simulink model "Problem1"  (R2020b)
settings: Solver=VariableStepAuto  StartTime=0.0  StopTime=10.0  RelTol=1e-3
settings Model: Creator=HP  LastModifiedBy=HP

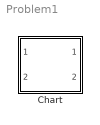
== system Problem1 ==
  Chart : Stateflow chart  TreatAsAtomicUnit=on

== stateflow chart Problem1/Chart ==
  state error
  state Coin_Inserted
  state Coke
  state Soda
  state Sprite
  state Pepsi
  (junction 5) -> error [order 2] : [money_insert<18]{Dispense=0}
  (default) -> Coin_Inserted
  Coin_Inserted -> error [order 1] : [money_insert<=0]{Dispense=0}
  Coin_Inserted -> (junction 5) [order 2] : [Drink_select==1]
  (junction 5) -> Coke [order 1] : [money_insert>=18]{Dispense=1, Diff_Amount=money_insert-18}
  (junction 12) -> error [order 2] : [money_insert<22]{Dispense=0}
  (junction 24) -> error [order 2] : [money_insert<20]{Dispense=0}
  (junction 23) -> error [order 2] : [money_insert<15]{Dispense=0}
  Coin_Inserted -> (junction 23) [order 4] : [Drink_select==3]
  Coin_Inserted -> (junction 24) [order 3] : [Drink_select==2]
  Coin_Inserted -> (junction 12) [order 5] : [Drink_select==4]
  (junction 23) -> Soda [order 1] : [money_insert>=15]{Dispense=1, Diff_Amount=money_insert-15}
  (junction 12) -> Sprite [order 1] : [money_insert>=22]{Dispense=1, Diff_Amount=money_insert-22}
  (junction 24) -> Pepsi [order 1] : [money_insert>=20]{Dispense=1, Diff_Amount=money_insert-20}
  data: Drink_select input; money_insert input; Diff_Amount output; Dispense output
